simulink model "Simulation"  (R2023b)
settings: Solver=ode4  StartTime=0.0  StopTime=Te  FixedStep=Ts/20  RelTol=1e-3
undefined symbols (not defined in the file): EgoCar1_params, egoCarID1, targetSpeed, Ts
libraries: drivingscenarioandsensors x7, trackingutilitieslib x2, drivinglib x1, sensorinslib x1
(part 3 of 6)

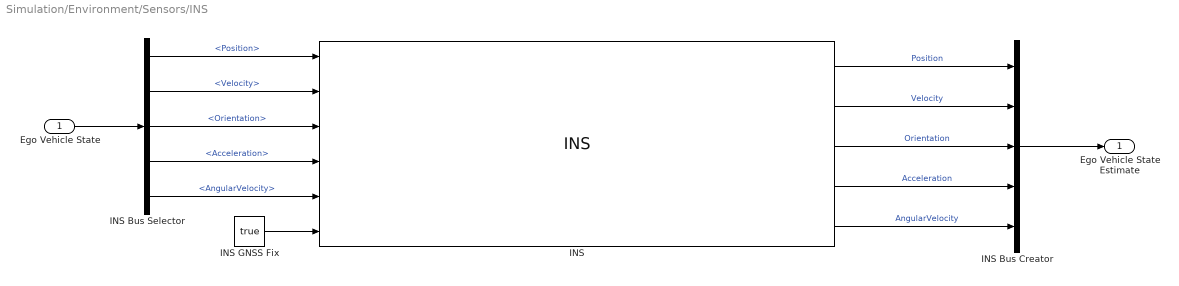
== system Simulation/Environment/Sensors/INS ==
  Ego Vehicle State : Inport
  INS : sensorinslib/INS  MountingLocation=[0 0 0]  RollAccuracy=EgoCar1_params.Sensors.INS.angleAccuraccy  PitchAccuracy=EgoCar1_params.Sensors.INS.angleAccuraccy  YawAccuracy=EgoCar1_params.Sensors.INS.angleAccuraccy  PositionAccuracy=[EgoCar1_params.Sensors.INS.positionAccuracy EgoCar1_params.Sensors.INS.positionAccuracy EgoCar1_params.Sensors.INS.positionAccuracy]  VelocityAccuracy=EgoCar1_params.Sensors.INS.angleAccuraccy  UseAccelAndAngVel=on  AccelerationAccuracy=0  AngularVelocityAccuracy=0  TimeInput=on  PositionErrorFactor=[0 0 0]  SeedDouble=67  SimulateUsing=Code generation
      settings: LibrarySourceBlock=drivingscenarioandsensors/INS
  INS Bus Creator : BusCreator  Inputs=5
  INS Bus Selector : BusSelector  OutputSignals=Position,Velocity,Orientation,Acceleration,AngularVelocity
  INS GNSS Fix : Constant  Value=true
  Ego Vehicle State Estimate : Outport
  wires:
  Ego Vehicle State/1 -> INS Bus Selector/1
  INS Bus Selector/2 -> INS/2  "<Velocity>"
  INS Bus Selector/4 -> INS/4  "<Acceleration>"
  INS Bus Selector/1 -> INS/1  "<Position>"
  INS/2 -> INS Bus Creator/2  "Velocity"
  INS/3 -> INS Bus Creator/3  "Orientation"
  INS Bus Selector/3 -> INS/3  "<Orientation>"
  INS/1 -> INS Bus Creator/1  "Position"
  INS Bus Selector/5 -> INS/5  "<AngularVelocity>"
  INS/4 -> INS Bus Creator/4  "Acceleration"
  INS Bus Creator/1 -> Ego Vehicle State Estimate/1
  INS/5 -> INS Bus Creator/5  "AngularVelocity"
  INS GNSS Fix/1 -> INS/6
